simulink model "Li_CellBalancing"  (R2025a)
settings: Solver=VariableStepAuto  StartTime=0.0  StopTime=inf  RelTol=1e-3
undefined symbols (not defined in the file): Ion, Lithium
libraries: spsBatteryLib x3, spsIdealSwitchLib x3, spsSeriesRLCLoadLib x3, spsVoltageMeasurementLib x1, sps_lib x1
settings Model: Creator=Dell  LastModifiedBy=Dell

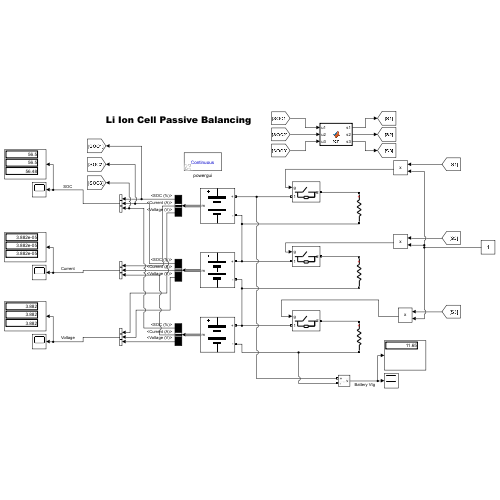
[thumbnail: Simulink's stored preview of the top-level diagram]
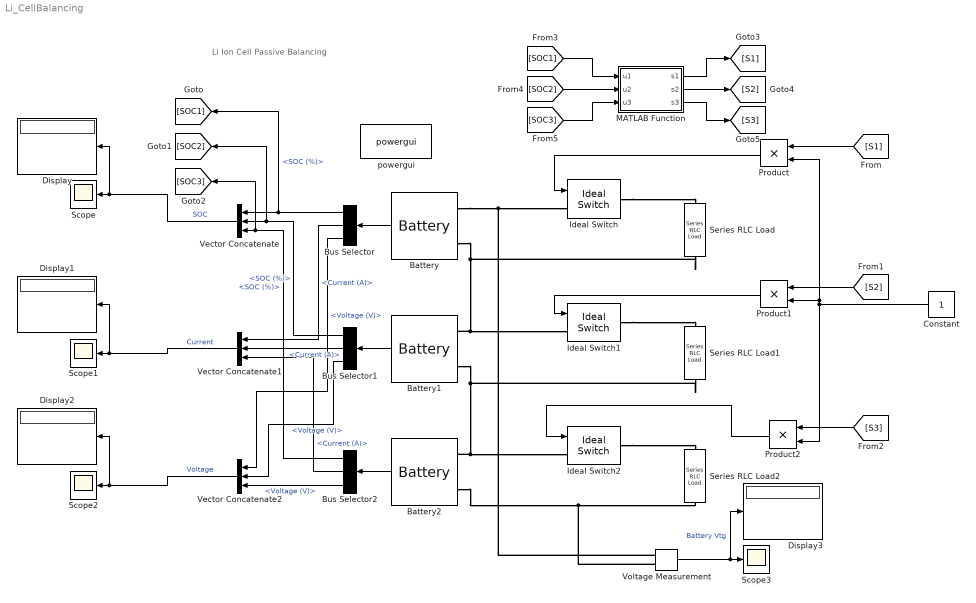
== system Li_CellBalancing ==
  note: Li Ion Cell Passive Balancing
  Battery : spsBatteryLib/Battery  BatType=Lithium-Ion  NomV=3.6  NomQ=250  SOC=85  Batt_Tr=.5  PresetModel=on  MaxQ=250  MinV=2.7  FullV=4.1904  Dis_rate=108.6957  R=0.000144  Normal_OP=226.087  expZone="[3.88939      12.2826]"
  Battery1 : spsBatteryLib/Battery  BatType=Lithium-Ion  NomV=3.6  NomQ=250  SOC=75  Batt_Tr=.5  PresetModel=on  MaxQ=250  MinV=2.7  FullV=4.1904  Dis_rate=108.6957  R=0.000144  Normal_OP=226.087  expZone="[3.88939      12.2826]"
  Battery2 : spsBatteryLib/Battery  BatType=Lithium-Ion  NomV=3.6  NomQ=250  SOC=55  Batt_Tr=.5  PresetModel=on  MaxQ=250  MinV=2.7  FullV=4.1904  Dis_rate=108.6957  R=0.000144  Normal_OP=226.087  expZone="[3.88939      12.2826]"
  Bus Selector : BusSelector  OutputSignals=SOC (%),Current (A),Voltage (V)
  Bus Selector1 : BusSelector  OutputSignals=SOC (%),Current (A),Voltage (V)
  Bus Selector2 : BusSelector  OutputSignals=SOC (%),Current (A),Voltage (V)
  Constant : Constant
  Display{,1..3} (4 alike) : Display
  Ideal Switch : spsIdealSwitchLib/Ideal Switch  Ron=0.001  Lon=0  IC=0  Rs=1e5  Cs=inf  Measurements=off
  Ideal Switch1 : spsIdealSwitchLib/Ideal Switch  Ron=0.001  Lon=0  IC=0  Rs=1e5  Cs=inf  Measurements=off
  Ideal Switch2 : spsIdealSwitchLib/Ideal Switch  Ron=0.001  Lon=0  IC=0  Rs=1e5  Cs=inf  Measurements=off
  MATLAB Function : MATLAB Function  TreatAsAtomicUnit=on
  Product : Product
  Product1 : Product
  Product2 : Product
  Scope{,1..3} (4 alike) : Scope
      Scope settings: SampleTime=100  TimeUnits=Metric (based on Time Span)  ActiveDisplayYMinimum=40.285856529644107  ActiveDisplayYMaximum=110.44472033513797
      Scope1 settings: ActiveDisplayYMinimum=-1  ActiveDisplayYMaximum=1
      Scope2 settings: ActiveDisplayYMinimum=-1  ActiveDisplayYMaximum=1  DataLoggingVariableName=ScopeData2
      Scope3 settings: DataLoggingVariableName=ScopeData3
  Series RLC Load : spsSeriesRLCLoadLib/Series RLC Load  LConnTagsString=a  RConnTagsString=__new0  NominalVoltage=3.6  NominalFrequency=60  ActivePower=1000  InductivePower=0  CapacitivePower=0  Setx0=off  InitialVoltage=0  SetiL0=off  InitialCurrent=0  Measurements=None  LoadType=constant Z
  Series RLC Load1 : spsSeriesRLCLoadLib/Series RLC Load  LConnTagsString=a  RConnTagsString=__new0  NominalVoltage=3.6  NominalFrequency=60  ActivePower=1000  InductivePower=0  CapacitivePower=0  Setx0=off  InitialVoltage=0  SetiL0=off  InitialCurrent=0  Measurements=None  LoadType=constant Z
  Series RLC Load2 : spsSeriesRLCLoadLib/Series RLC Load  LConnTagsString=a  RConnTagsString=__new0  NominalVoltage=3.6  NominalFrequency=60  ActivePower=1000  InductivePower=0  CapacitivePower=0  Setx0=off  InitialVoltage=0  SetiL0=off  InitialCurrent=0  Measurements=None  LoadType=constant Z
  Vector Concatenate : Concatenate  NumInputs=3
  Vector Concatenate1 : Concatenate  NumInputs=3
  Vector Concatenate2 : Concatenate  NumInputs=3
  Voltage Measurement : spsVoltageMeasurementLib/Voltage Measurement  PhasorSimulation=off  OutputType=Complex  PSBequivalent=0
  powergui : sps_lib/powergui  Priority=1  SimulationMode=Continuous  SampleTime=50e-6  frequency=60  Iterations=50  frequencyindice=0  Pbase=100e6  ErrMax=1e-4  UnitsV=kV  UnitsW=MW  buscounter=0  FunctionMessages=off  echomessages=off  EnableUseOfTLC=off  CurrentSourceSwitches=off  DisableSnubberDevices=off  DisableRonSwitches=off  DisableVfSwitches=off  DisplayEquations=off  AutomaticDiscreteSolvers=off  SolverType=Tustin/Backward Euler (TBE)  Interpol=off  ExternalGateDelay=off  methode=off  Ts=100  x0status=blocks  SPID=on  SwTol=0  HookPort=off  NonlinearTolerance=1e-4  nMaxIteration=100  ContinueOnMaxIteration=off  RestoreLinks=warning  ResistiveCurrentMeasurement=off  Frange=[0:2:500]  Ylog=off  Xlog=on  ShowGrid=off  save=off  variable=ZData  structure=0  ZoomFFT=off  StartTime=0.0  cycles=1  DisplayStyle=1  fundamental=60  FreqAxis=off  MaxFrequency=1000  frequencyindicesteady=1  RmsSteady=1  display=off
  wires:
  Product/1 -> Ideal Switch/1
  Product1/1 -> Ideal Switch1/1
  Product2/1 -> Ideal Switch2/1
  Constant/1 -> Product1/2, Product/2, Product2/2
  [S1] -> Product/1
  [S2] -> Product1/1
  [S3] -> Product2/1
  Battery/1 -> Bus Selector/1
  Battery1/1 -> Bus Selector1/1
  Battery2/1 -> Bus Selector2/1
  Bus Selector/1 -> Vector Concatenate/1, [SOC1]  "<SOC (%)>"
  Bus Selector1/1 -> Vector Concatenate/2, [SOC2]  "<SOC (%)>"
  Bus Selector2/1 -> [SOC3], Vector Concatenate/3  "<SOC (%)>"
  Bus Selector1/2 -> Vector Concatenate1/2  "<Current (A)>"
  Bus Selector/2 -> Vector Concatenate1/1  "<Current (A)>"
  Bus Selector2/2 -> Vector Concatenate1/3  "<Current (A)>"
  Bus Selector/3 -> Vector Concatenate2/1  "<Voltage (V)>"
  Bus Selector1/3 -> Vector Concatenate2/2  "<Voltage (V)>"
  Bus Selector2/3 -> Vector Concatenate2/3  "<Voltage (V)>"
  Vector Concatenate/1 -> Display/1, Scope/1  "SOC"
  Vector Concatenate1/1 -> Display1/1, Scope1/1  "Current"
  Vector Concatenate2/1 -> Display2/1, Scope2/1  "Voltage"
  Voltage Measurement/1 -> Display3/1, Scope3/1  "Battery Vtg"
  [SOC2] -> MATLAB Function/2(u2)
  [SOC1] -> MATLAB Function/1(u1)
  [SOC3] -> MATLAB Function/3(u3)
  MATLAB Function/1(s1) -> [S1]
  MATLAB Function/2(s2) -> [S2]
  MATLAB Function/3(s3) -> [S3]
  connections:
  Battery/LConn2 -- Series RLC Load/RConn1 -- Ideal Switch1/LConn1 -- Battery1/LConn1
  Battery1/LConn2 -- Series RLC Load1/RConn1 -- Ideal Switch2/LConn1 -- Battery2/LConn1
  Battery/LConn1 -- Voltage Measurement/LConn1 -- Ideal Switch/LConn1
  Ideal Switch/RConn1 -- Series RLC Load/LConn1
  Ideal Switch1/RConn1 -- Series RLC Load1/LConn1
  Ideal Switch2/RConn1 -- Series RLC Load2/LConn1
  Battery2/LConn2 -- Voltage Measurement/LConn2 -- Series RLC Load2/RConn1

== matlab function Li_CellBalancing/MATLAB Function ==
  data: u1 input; s1 output; u2 input; u3 input; s2 output; s3 output
function [s1,s2,s3] = fcn(u1,u2,u3)

u1 = int32(u1);
u2 = int32(u2);
u3 = int32(u3);

if ((u1>u2)||(u1>u3))
    s1 = 1;    
else
    s1 = 0;
end
    if ((u2>u1)||(u2>u3))
        s2 = 1;    
    else
        s2 = 0;
    end
        if ((u3>u1)||(u3>u2))
            s3 = 1;
        else
            s3 = 0;
        end
